simulink model "final_output"  (R2024a)
settings: Solver=VariableStepAuto  StartTime=0.0  StopTime=2  MaxStep=1e-3  RelTol=1e-3  EnableMultiTasking=on
PreLoadFcn:
  | DualActiveBridgeConverterData
values from neighbouring files (symbols this model uses):
  C_HV = 0.0001    [matlab.mat]
  C_LV = 0.002    [matlab.mat]
  Cs_FET = inf    [matlab.mat]
  Fsw = 100000    [matlab.mat]
  Ki_Ireg = 500    [matlab.mat]
  Kp_Ireg = 0.1    [matlab.mat]
  L_Inductor = 1.5e-05    [matlab.mat]
  Lm_Tr = 0.00072    [matlab.mat]
  Lprim_Tr = 1.7e-05    [matlab.mat]
  Lsec_Tr = 0    [matlab.mat]
  N_Tr = 1.6    [matlab.mat]
  Pnom = 10000    [matlab.mat]
  R_DCsrc1 = 0.01    [matlab.mat]
  R_DCsrc2 = 0.05    [matlab.mat]
  R_Inductor = 0.016    [matlab.mat]
  RC_HV = 0.001    [matlab.mat]
  RC_LV = 0.001    [matlab.mat]
  Rm_Tr = 10000    [matlab.mat]
  Ron_Diode = 0.01    [matlab.mat]
  Ron_FET = 0.016    [matlab.mat]
  Rprim_Tr = 0.043    [matlab.mat]
  Rs_FET = 1000000    [matlab.mat]
  Rsec_Tr = 1e-06    [matlab.mat]
  Ts_Control = 1e-06    [matlab.mat]
  Vf_Diode = 4.2    [matlab.mat]
  Vnom_HV = 800    [matlab.mat]
  Vnom_LV = 450    [matlab.mat]
undefined symbols (not defined in the file or in its folder): DiscIntNeverNeededParam, Ion, Lithium
libraries: spsSeriesRLCBranchLib x14, spsDiodeLib x12, spsVoltageMeasurementLib x11, spsMosfetLib x9, spsCurrentMeasurementLib x8, spsIdealSwitchLib x8, powerlib_extras x5, spsMeanLib x5, spsRMSLib x3, simulink x3, spsThreePhaseVIMeasurementLib x2, spsUniversalBridgeLib x2
(part 1 of 2)
settings Model: SimulationMode=accelerator  Creator=The MathWorks, Inc.  LastModifiedBy=suchi
settings SolverCC: ZeroCrossAlgorithm=Adaptive  AlgebraicLoopSolver=TrustRegion
settings DataIOCC: LimitDataPoints=on  SaveFormat=Array  SaveOutput=off  DSMLogging=off  SaveTime=off  ReturnWorkspaceOutputs=off
settings OptimizationCC: LifeSpan=inf
settings DebuggingCC: SaveWithParameterizedLinksMsg=none  UnderspecifiedInitializationDetection=Classic  MergeDetectMultiDrivingBlocksExec=none  IgnoredZcDiagnostic=none  SolverPrmCheckMsg=warning  FcnCallInpInsideContextMsg=warning  UnconnectedInputMsg=warning  UnconnectedOutputMsg=warning  UnconnectedLineMsg=warning  StateNameClashWarn=warning  SubsystemReferenceDiagnosticForUnitTest=warning  SFUnexpectedBacktrackingDiag=warning  SFNoUnconditionalDefaultTransitionDiag=warning  SFExecutionAtInitializationDiag=none  ArithmeticOperatorsInVariantConditions=warning
settings HardwareCC: ProdBitPerPointer=32  ProdBitPerSizeT=32  ProdBitPerPtrDiffT=32  ProdLargestAtomicFloat=None  ProdIntDivRoundTo=Undefined  ProdEndianess=Unspecified  ProdWordSize=32  ProdHWDeviceType=32-bit Generic  TargetHWDeviceType=32-bit Generic
settings ModelReferenceCC: EnableRefExpFcnMdlSchedulingChecks=on  PropagateSignalLabelsOutOfModel=off
settings SFSimCC: SimUseLocalCustomCode=off  CustomCodeUndefinedFunction=UseInterfaceOnly
settings RTWCC: RTWUseLocalCustomCode=off  GPUComputeCapability=3.5  DLArmComputeVersion=19.05
settings CodeAppCC: StateflowObjectComments=on
settings GRTTargetCC: TargetFcnLib=ansi_tfl_tmw.mat  TargetLangStandard=C89/C90 (ANSI)  CombineOutputUpdateFcns=off  GRTInterface=on
settings ConfigComp: CovMetricSettings=dw  CovSaveCumulativeToWorkspaceVar=on  CovSaveSingleToWorkspaceVar=on  CovExternalEMLEnable=off  CovSFcnEnable=off

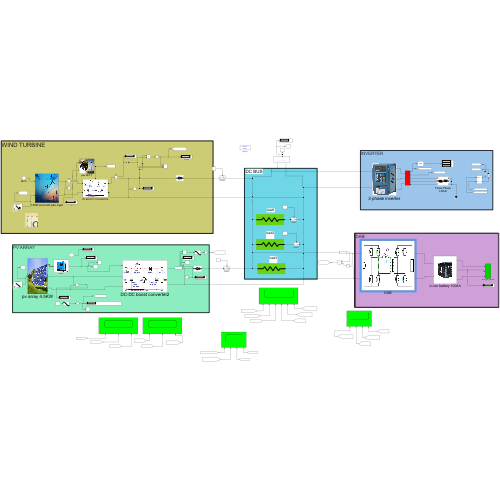
[thumbnail: Simulink's stored preview of the top-level diagram]
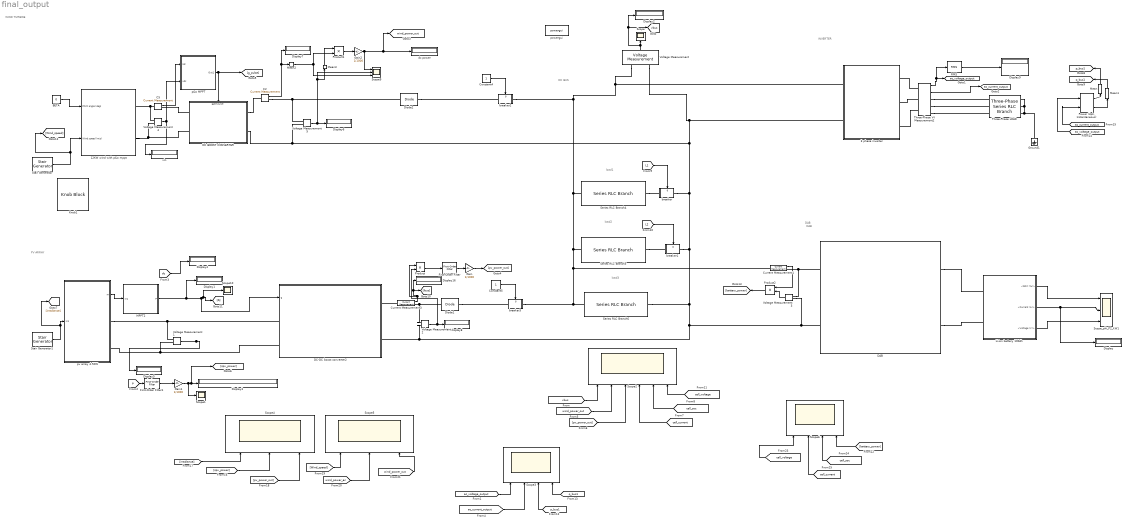
== system final_output ==
  note: DC BUS
  note: load1
  note: INVERTER
  note: DAB
  note: WIND TURBINE
  note: PV ARRAY
  note: load3
  note: load2
  note: DAB
  12KW wind with p&o mppt : Subsystem
      mask Display: image('download (1) - Copy.jpeg');
  3 phase inverter : Subsystem
      mask Display: image('63494ce6710fec25d6700b0f-vfd-inverter-ac-380v-4kw-three-phase.jpg');
  BETA : Constant  Value=0
  C2 : spsCurrentMeasurementLib/Current Measurement  PhasorSimulation=off  OutputType=Complex  PSBequivalent=0
  C5 : spsCurrentMeasurementLib/Current Measurement  PhasorSimulation=off  OutputType=Complex  PSBequivalent=0
  Constant4 : Constant
  Constant5 : Constant
  Current Measurement1 : spsCurrentMeasurementLib/Current Measurement  PhasorSimulation=off  OutputType=Complex  PSBequivalent=0
  Current Measurement3 : spsCurrentMeasurementLib/Current Measurement  PhasorSimulation=off  OutputType=Complex  PSBequivalent=0
  DAB : Subsystem
      mask Display: image('DAB.jpg');
  DC BOOST CONVERTER : Subsystem
      settings: PortSchema="{\"entries\":[{\"content\":{\"sides\":[{\"content\":{\"connectorIds\":[\"LConn1\",\"LConn2\"]},\"type\":\"ConnectorPlacement.EquallySpacedRectSide\",\"uuid\":\"56be2a4d-d0e9-492c-96c1-3864bac83254\"},{\"content\":{\"connectorIds\":[\"RConn1\",\"RConn2\"],\"side\":\"RIGHT\"},\"type\":\"ConnectorPlacement.EquallySpacedRectSide\",\"uuid\":\"94a95191-bdc4-49b6-9a1b-7d416a9cf8d0\"},{\"content\":{\"connectorIds\":[\"In1\"],\"side\":\"TOP\"},\"type\":\"ConnectorPlacement.EquallySpacedRectSide\",\"uuid\":\"679d3c69-2a7c-41fc-a2c8-ece2ac62cc84\"}]},\"type\":\"ConnectorPlacement.EquallySpacedConnector\",\"uuid\":\"33c0da2b-e95a-43d2-a39b-7409ff7da8a9\"}],\"packageUris\":[\"http://schema.mathworks.com/mf0/Connector/R2020b\"],\"version\":\"1.0\"}"
      mask Display: image('boost-converter-working-model.jpg');
  DC-DC boost converter2 : Subsystem
      mask Display: image('boost-converter-working-model.jpg');
  Diode1 : spsDiodeLib/Diode  Ron=0.001  Lon=0  Vf=0.8  IC=0  UseSnubber=0  Rs=inf  Cs=250e-9  Measurements=off
  Diode2 : spsDiodeLib/Diode  Ron=0.001  Lon=0  Vf=0.8  IC=0  UseSnubber=0  Rs=inf  Cs=250e-9  Measurements=off
  Display{,1..9,16} (11 alike) : Display
  First-Order Filter : spsFirstOrderFilterLib/First-Order Filter  FilterType=Lowpass  Tc=10e-3  Ts=0  Initialize=on  Vac_Init=[0, 0, 60]  Vdc_Init=0  PlotResponse=off  FreqRange="[0,  200,  1]"
  First-Order Filter1 : spsFirstOrderFilterLib/First-Order Filter  FilterType=Lowpass  Tc=10e-3  Ts=0  Initialize=on  Vac_Init=[0, 0, 60]  Vdc_Init=0  PlotResponse=off  FreqRange="[0,  200,  1]"
  Gain : Gain  Gain=1/1000
  Gain1 : Gain  Gain=1/1000
  Gain2 : Gain  Gain=1/1000
  Goto11 : Goto
  Ground1 : spsGroundLib/Ground  LConnTagsString=a
  Knob1 : KnobBlock  ScaleMax=20
  Li-ion battery 100Ah : Subsystem
      mask Display: image('Lion-Adventure-side-2000x2000 (1).png');
  MPPT2 : Subsystem
      mask Display: image('48v-50a-mppt-solar-charge-.png');
  Mean : spsMeanLib/Mean  Freq=50  Vinit=0  Ts=0
  Mean1 : spsMeanLib/Mean  Freq=50  Vinit=0  Ts=0
  Mean2 : spsMeanLib/Mean  Freq=50  Vinit=0  Ts=50e-6
  Mean3 : spsMeanLib/Mean  Freq=50  Vinit=0  Ts=50e-6
  "Power (3ph, Instantaneous)" : spsPower3phInstantaneousLib/Power (3ph, Instantaneous)
  Product : Product
  Product1 : Product
  Product2 : Product
  RMS : spsRMSLib/RMS  TrueRMS=on  Freq=50  RMSInit=120  Ts=0
  Scope : Scope
  Scope1 : Scope
  Scope10 : Scope
  Scope2 : Scope  NumInputPorts=6
  Scope3 : Scope  NumInputPorts=4
  Scope4 : Scope  NumInputPorts=3
  Scope5 : Scope  NumInputPorts=3
  Scope6 : Scope  NumInputPorts=4
  Scope9 : Scope  NumInputPorts=3
  Scope_phi_P2_kW1 : Scope  NumInputPorts=3
  Series RLC Branch4 : spsSeriesRLCBranchLib/Series RLC Branch  LConnTagsString=__new0  RConnTagsString=__new0  BranchType=R  Resistance=100  Inductance=1e-9  SetiL0=off  InitialCurrent=0  Capacitance=10  Setx0=off  InitialVoltage=0  Measurements=None
  Series RLC Branch5 : spsSeriesRLCBranchLib/Series RLC Branch  LConnTagsString=__new0  RConnTagsString=__new0  BranchType=R  Resistance=100  Inductance=1e-9  SetiL0=off  InitialCurrent=0  Capacitance=10  Setx0=off  InitialVoltage=0  Measurements=None
  Series RLC Branch6 : spsSeriesRLCBranchLib/Series RLC Branch  LConnTagsString=__new0  RConnTagsString=__new0  BranchType=R  Resistance=120  Inductance=1e-9  SetiL0=off  InitialCurrent=0  Capacitance=10  Setx0=off  InitialVoltage=0  Measurements=None
  Stair Generator : eeStairGenerator/Stair Generator  LabelModeActiveChoice=Discrete  TimeInput=[0 0.4 0.8 1.2 1.4 1.6 1.8 ]  AmplitudeInput=[12 10 8 6 8 10 6 ]  SampleTime=-1  RepeatPattern=off  OutDataTypeStr=double
      settings: LibrarySourceBlock=ee_sl_lib/General Control/Stair Generator
  Stair Generator1 : eeStairGenerator/Stair Generator  LabelModeActiveChoice=Discrete  TimeInput=[0 0.4 0.8 1.2 1.6 1.8 ]  AmplitudeInput=[1000 800 600 400 200 400]  SampleTime=1e-6  RepeatPattern=off  OutDataTypeStr=double
      settings: LibrarySourceBlock=ee_sl_lib/General Control/Stair Generator
  Three-Phase LOAD : spsThreePhaseSeriesRLCBranchLib/Three-Phase Series RLC Branch  LConnTagsString=A|B|C  RConnTagsString=A|B|C  BranchType=RL  Resistance=100  Inductance=100e-3  Capacitance=1e-6  Measurements=None
  Three-Phase V-I Measurement2 : spsThreePhaseVIMeasurementLib/Three-Phase V-I Measurement  VoltageMeasurement=phase-to-phase  SetLabelV=off  LabelV=Vabc  Vpu=off  VpuLL=off  CurrentMeasurement=yes  SetLabelI=off  LabelI=Iabc  Ipu=off  Pbase=100e6  Vbase=500e3  OutputType=Complex  PhasorSimulation=off  PSBequivalent=0
  Voltage Measurement{,1..5} (6 alike) : spsVoltageMeasurementLib/Voltage Measurement  PhasorSimulation=off  OutputType=Complex  PSBequivalent=0
  breaker : Subsystem
      settings: PortSchema="{\"entries\":[{\"content\":{\"sides\":[{\"content\":{\"connectorIds\":[\"LConn1\"]},\"type\":\"ConnectorPlacement.EquallySpacedRectSide\",\"uuid\":\"d9a674fe-e63c-428a-8f68-a3d0edc2d0cb\"},{\"content\":{\"connectorIds\":[\"RConn1\"],\"side\":\"RIGHT\"},\"type\":\"ConnectorPlacement.EquallySpacedRectSide\",\"uuid\":\"8621f35b-529d-46ae-a8cf-f4891c99fec3\"},{\"content\":{\"connectorIds\":[\"In1\"],\"side\":\"TOP\"},\"type\":\"ConnectorPlacement.EquallySpacedRectSide\",\"uuid\":\"fecd911f-8796-40e3-a2af-44f182b78dc1\"}]},\"type\":\"ConnectorPlacement.EquallySpacedConnector\",\"uuid\":\"73397587-ab48-451b-aa61-cf3e3594506e\"}],\"packageUris\":[\"http://schema.mathworks.com/mf0/Connector/R2020b\"],\"version\":\"1.0\"}"
  breaker1 : Subsystem
      settings: PortSchema="{\"entries\":[{\"content\":{\"sides\":[{\"content\":{\"connectorIds\":[\"LConn1\"]},\"type\":\"ConnectorPlacement.EquallySpacedRectSide\",\"uuid\":\"d9a674fe-e63c-428a-8f68-a3d0edc2d0cb\"},{\"content\":{\"connectorIds\":[\"RConn1\"],\"side\":\"RIGHT\"},\"type\":\"ConnectorPlacement.EquallySpacedRectSide\",\"uuid\":\"8621f35b-529d-46ae-a8cf-f4891c99fec3\"},{\"content\":{\"connectorIds\":[\"In1\"],\"side\":\"TOP\"},\"type\":\"ConnectorPlacement.EquallySpacedRectSide\",\"uuid\":\"fecd911f-8796-40e3-a2af-44f182b78dc1\"},{\"content\":{\"side\":\"BOTTOM\"},\"type\":\"ConnectorPlacement.EquallySpacedRectSide\",\"uuid\":\"1105760b-ea89-4923-b494-35b0f35b7535\"}]},\"type\":\"ConnectorPlacement.EquallySpacedConnector\",\"uuid\":\"73397587-ab48-451b-aa61-cf3e3594506e\"}],\"packageUris\":[\"http://schema.mathworks.com/mf0/Connector/R2020b\"],\"version\":\"1.0\"}"
  breaker2 : Subsystem
      settings: PortSchema="{\"entries\":[{\"content\":{\"sides\":[{\"content\":{\"connectorIds\":[\"LConn1\"]},\"type\":\"ConnectorPlacement.EquallySpacedRectSide\",\"uuid\":\"d9a674fe-e63c-428a-8f68-a3d0edc2d0cb\"},{\"content\":{\"connectorIds\":[\"RConn1\"],\"side\":\"RIGHT\"},\"type\":\"ConnectorPlacement.EquallySpacedRectSide\",\"uuid\":\"8621f35b-529d-46ae-a8cf-f4891c99fec3\"},{\"content\":{\"connectorIds\":[\"In1\"],\"side\":\"TOP\"},\"type\":\"ConnectorPlacement.EquallySpacedRectSide\",\"uuid\":\"fecd911f-8796-40e3-a2af-44f182b78dc1\"}]},\"type\":\"ConnectorPlacement.EquallySpacedConnector\",\"uuid\":\"73397587-ab48-451b-aa61-cf3e3594506e\"}],\"packageUris\":[\"http://schema.mathworks.com/mf0/Connector/R2020b\"],\"version\":\"1.0\"}"
  breaker3 : Subsystem
      settings: PortSchema="{\"entries\":[{\"content\":{\"sides\":[{\"content\":{\"connectorIds\":[\"LConn1\"]},\"type\":\"ConnectorPlacement.EquallySpacedRectSide\",\"uuid\":\"d9a674fe-e63c-428a-8f68-a3d0edc2d0cb\"},{\"content\":{\"connectorIds\":[\"RConn1\"],\"side\":\"RIGHT\"},\"type\":\"ConnectorPlacement.EquallySpacedRectSide\",\"uuid\":\"8621f35b-529d-46ae-a8cf-f4891c99fec3\"},{\"content\":{\"connectorIds\":[\"In1\"],\"side\":\"TOP\"},\"type\":\"ConnectorPlacement.EquallySpacedRectSide\",\"uuid\":\"fecd911f-8796-40e3-a2af-44f182b78dc1\"}]},\"type\":\"ConnectorPlacement.EquallySpacedConnector\",\"uuid\":\"73397587-ab48-451b-aa61-cf3e3594506e\"}],\"packageUris\":[\"http://schema.mathworks.com/mf0/Connector/R2020b\"],\"version\":\"1.0\"}"
  dc power : Display
  p&o MPPT : Subsystem
      mask Display: image('Wind-Turbine-MPPT-Charge-Controller (1).png');
  powergui : sps_lib/powergui  Priority=1  SimulationMode=Discrete  SampleTime=1e-6  frequency=60  Iterations=50  frequencyindice=0  Pbase=100e6  ErrMax=1e-4  UnitsV=kV  UnitsW=MW  buscounter=0  FunctionMessages=off  echomessages=off  EnableUseOfTLC=off  CurrentSourceSwitches=off  DisableSnubberDevices=off  DisableRonSwitches=off  DisableVfSwitches=off  DisplayEquations=off  AutomaticDiscreteSolvers=off  SolverType=Tustin/Backward Euler (TBE)  Interpol=off  ExternalGateDelay=off  methode=off  Ts=100  x0status=blocks  SPID=on  SwTol=0  HookPort=off  NonlinearTolerance=1e-4  nMaxIteration=100  ContinueOnMaxIteration=off  RestoreLinks=warning  ResistiveCurrentMeasurement=off  Frange=[0:2:500]  Ylog=off  Xlog=on  ShowGrid=off  save=off  variable=ZData  structure=0  ZoomFFT=off  StartTime=0.0  cycles=1  DisplayStyle=1  fundamental=60  FreqAxis=off  MaxFrequency=1000  frequencyindicesteady=1  RmsSteady=1  display=off
  pv array 4.5KW : Subsystem
      mask Display: image('shutterstock-630302630-solar-panel-dealers-2-i44i3.png');
  vin : Display
  tag scope: ac_current_output=global, ac_voltage_output=global, p_bus1=global, q_bus1=global, vbus=global, wind_power_out=global
  wires:
  Stair Generator1/1 -> [irradiance], pv array 4.5KW/1(In1)
  pv array 4.5KW/1(m) -> MPPT2/1(In1)
  MPPT2/1(P) -> Display1/1, Goto11/1, Scope10/1, DC-DC boost converter2/1(g)
  Current Measurement3/1 -> Product/1, Display16/1, [ibus]
  [dc] -> Display4/1
  Voltage Measurement1/1 -> Display5/1
  RMS/1 -> Display9/1
  Three-Phase V-I Measurement2/1 -> RMS/1, [ac_voltage_output]
  Three-Phase V-I Measurement2/2 -> [ac_current_output]
  [L1] -> breaker/1(g)
  [L2] -> breaker1/1(g)
  Li-ion battery 100Ah/2(<Current (A)>) -> Display/1, Scope_phi_P2_kW1/2
  Li-ion battery 100Ah/1(<SOC (%)>) -> Scope_phi_P2_kW1/1
  Li-ion battery 100Ah/3(<Voltage (V)>) -> Scope_phi_P2_kW1/3
  Voltage Measurement/1 -> [vbus], Display2/1, Scope/1
  BETA/1 -> 12KW wind with p&o mppt/1(Pitch angle (deg))
  Voltage Measurement5/1 -> Display6/1, Mean3/1, Scope9/2
  Mean3/1 -> Product1/1
  Gain2/1 -> Scope9/1, [wind_power_out], dc power/1
  Mean2/1 -> Product1/2, Scope9/3
  C2/1 -> Display7/1, Mean2/1
  Product1/1 -> Gain2/1
  Voltage Measurement2/1 -> Product/2, Display8/1
  [vbus] -> Scope2/1
  [wind_power_out] -> Scope2/2
  Product/1 -> First-Order Filter/1
  [pv_power_out] -> Scope2/3
  Constant4/1 -> breaker2/1(g)
  Constant5/1 -> breaker3/1(g)
  First-Order Filter/1 -> Gain/1
  p&o MPPT/1(Out1) -> [g_pulse], DC BOOST CONVERTER/1(gate pulse)
  Voltage Measurement4/1 -> vin/1, p&o MPPT/2(vdc)
  C5/1 -> p&o MPPT/1(Idc)
  Gain/1 -> [pv_power_out]
  [p] -> First-Order Filter1/1
  First-Order Filter1/1 -> Gain1/1
  Gain1/1 -> Scope1/1, [spv_power], Display3/1
  [cell_current] -> Scope2/4
  [cell_soc] -> Scope2/5
  [cell_voltage] -> Scope2/6
  [ac_voltage_output] -> Scope3/1
  [ac_current_output] -> Scope3/2
  [p_bus1] -> Scope3/3
  [q_bus1] -> Scope3/4
  [ac_voltage_output] -> "Power (3ph, Instantaneous)"/1
  [ac_current_output] -> "Power (3ph, Instantaneous)"/2
  "Power (3ph, Instantaneous)"/1 -> Mean/1
  "Power (3ph, Instantaneous)"/2 -> Mean1/1
  Mean/1 -> [p_bus1]
  Mean1/1 -> [q_bus1]
  [irradiance] -> Scope4/1
  [spv_power] -> Scope4/2
  [pv_power_out] -> Scope4/3
  Stair Generator/1 -> [Wind_speed], 12KW wind with p&o mppt/2(Wind speed (m/s))
  [Wind_speed] -> Scope5/1
  [wind_power_ac] -> Scope5/2
  [wind_power_out] -> Scope5/3
  Voltage Measurement3/1 -> Product2/2
  Current Measurement1/1 -> Product2/1
  Product2/1 -> [battery_power]
  [cell_voltage] -> Scope6/1
  [battery_power] -> Scope6/4
  [cell_soc] -> Scope6/3
  [cell_current] -> Scope6/2
  connections:
  Current Measurement3/RConn1 -- Voltage Measurement2/LConn1 -- Diode1/LConn1
  DC-DC boost converter2/LConn2 -- Voltage Measurement1/LConn2 -- pv array 4.5KW/RConn2
  pv array 4.5KW/RConn1 -- Voltage Measurement1/LConn1 -- DC-DC boost converter2/LConn1
  Current Measurement3/LConn1 -- DC-DC boost converter2/RConn1
  Three-Phase LOAD/RConn1 -- Ground1/LConn1 -- Three-Phase LOAD/RConn3 -- Three-Phase LOAD/RConn2
  Three-Phase V-I Measurement2/LConn3 -- 3 phase inverter/LConn3
  Three-Phase V-I Measurement2/LConn1 -- 3 phase inverter/LConn1
  Three-Phase V-I Measurement2/RConn1 -- Three-Phase LOAD/LConn1
  Three-Phase V-I Measurement2/LConn2 -- 3 phase inverter/LConn2
  DAB/LConn1 -- Voltage Measurement3/LConn1 -- Current Measurement1/RConn1
  Series RLC Branch4/RConn1 -- breaker/LConn1
  Series RLC Branch5/RConn1 -- breaker1/LConn1
  DAB/RConn1 -- Li-ion battery 100Ah/LConn1
  DAB/RConn2 -- Li-ion battery 100Ah/LConn2
  Voltage Measurement5/LConn2 -- DC BOOST CONVERTER/RConn2 -- Voltage Measurement/LConn2 -- 3 phase inverter/RConn2 -- Voltage Measurement3/LConn2 -- DAB/LConn2 -- DC-DC boost converter2/RConn2 -- Voltage Measurement2/LConn2 -- Series RLC Branch6/RConn1 -- breaker1/RConn1 -- breaker/RConn1
  C2/RConn1 -- Voltage Measurement5/LConn1 -- Diode2/LConn1
  Diode2/RConn1 -- breaker2/LConn1
  Diode1/RConn1 -- breaker3/LConn1
  DC BOOST CONVERTER/RConn1 -- C2/LConn1
  12KW wind with p&o mppt/RConn2 -- Voltage Measurement4/LConn2 -- DC BOOST CONVERTER/LConn2
  C5/LConn1 -- Voltage Measurement4/LConn1 -- 12KW wind with p&o mppt/RConn1
  C5/RConn1 -- DC BOOST CONVERTER/LConn1
  Three-Phase V-I Measurement2/RConn2 -- Three-Phase LOAD/LConn2
  Three-Phase V-I Measurement2/RConn3 -- Three-Phase LOAD/LConn3
  Current Measurement1/LConn1 -- breaker3/RConn1 -- Series RLC Branch6/LConn1 -- Voltage Measurement/LConn1 -- 3 phase inverter/RConn1 -- breaker2/RConn1 -- Series RLC Branch4/LConn1 -- Series RLC Branch5/LConn1

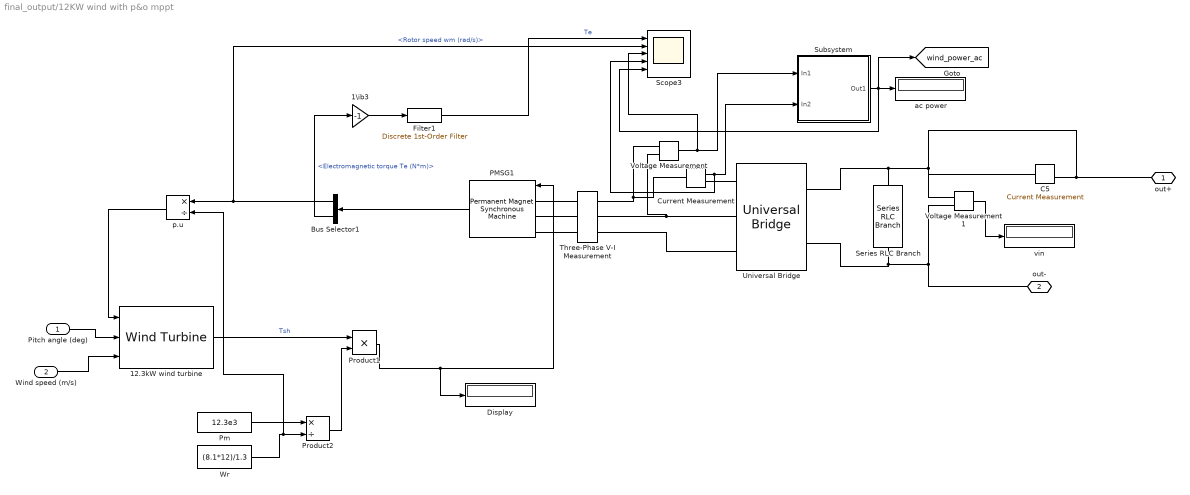
== system final_output/12KW wind with p&o mppt ==
  Pitch angle (deg) : Inport
  Wind speed (m/s) : Inport  Port=2
  "12.3kW wind turbine " : spsWindTurbineLib/Wind Turbine  Pnom=12.3e3  Pelec_base=12.3e3/0.9  wind_base=12  P_wind_base=0.85  speed_nom=1.2  pitch_angle=0  c1_c6="[0.51763          116          0.4            5           21     0.006795]"  cp_nom=0.48  lambda_nom=8.1
  1\ib3 : Gain  Gain=-1  SaturateOnIntegerOverflow=on  OutDataTypeStr=Inherit: Same as input  ParamDataTypeStr=Inherit: Same as input
  Bus Selector1 : BusSelector  OutputSignals=Rotor speed wm (rad/s),Electromagnetic torque Te (N*m)
  C5 : spsCurrentMeasurementLib/Current Measurement  PhasorSimulation=off  OutputType=Complex  PSBequivalent=0
  Current Measurement : spsCurrentMeasurementLib/Current Measurement  PhasorSimulation=off  OutputType=Complex  PSBequivalent=0
  Display : Display
  Filter1 : powerlib_extras/Discrete  Control Blocks/Discrete 1st-Order Filter  FilterType=Lowpass  Tc=1e-3  Ts=50e-6  Initialize=off  Vac_Init=[0.8 -25 50]  Vdc_Init=-0.4  PlotResponse=off  param1=[1 500 0.1]
  PMSG1 : spsPermanentMagnetSynchronousMachineLib/Permanent Magnet Synchronous Machine  NbPhases=3  FluxDistribution=Sinusoidal  RotorType=Salient-pole  MechanicalLoad=Torque Tm  PresetModel=No  ShowDetailedParameters=on  MeasurementBus=off  Resistance=0.0485  Inductance=8.5e-3  dqInductances=[0.395e-3 0.395e-3]  La=0.000835  MachineConstant=Flux linkage established by magnets (V.s)  Flux=0.1194  VoltageCst=108.2838  TorqueCst=0.8955  Flat=120  Mechanical=[0.01197 0.001189 5]  PolePairs=5  InitialConditions=[0,0, 0,0]  InitialConditions5ph=[0 0 0 0 0 0]  RefAngle=90 degrees behind phase A axis (modified Park)  IterativeDiscreteModel=Trapezoidal non iterative  TsBlock=-1  TsPowergui=0
  Pm : Constant  Value=12.3e3
  Product1 : Product
  Product2 : Product  Inputs=*/
  Scope3 : Scope  NumInputPorts=5
  Series RLC Branch : spsSeriesRLCBranchLib/Series RLC Branch  LConnTagsString=__new0  RConnTagsString=__new0  BranchType=RC  Resistance=0.005  Inductance=1e-3  SetiL0=off  InitialCurrent=0  Capacitance=6.60937e-03  Setx0=off  InitialVoltage=0  Measurements=None
  Subsystem : Subsystem
  Three-Phase V-I Measurement : spsThreePhaseVIMeasurementLib/Three-Phase V-I Measurement  VoltageMeasurement=no  SetLabelV=off  LabelV=Vabc  Vpu=off  VpuLL=off  CurrentMeasurement=no  SetLabelI=off  LabelI=Iabc  Ipu=off  Pbase=100e6  Vbase=500e3  OutputType=Complex  PhasorSimulation=off  PSBequivalent=0
  Universal Bridge : spsUniversalBridgeLib/Universal Bridge  Arms=3  SnubberResistance=1e5  SnubberCapacitance=inf  Device=Diodes  Ron=1e-3  Lon=0  ForwardVoltages="[  0  0  ]"  ForwardVoltage=0  GTOparameters=[ 10e-6 , 20e-6 ]  IGBTparameters=[ 1e-6 , 2e-6 ]  Measurements=None  Measurements_2=None  converterType=Rectifier
  Voltage Measurement : spsVoltageMeasurementLib/Voltage Measurement  PhasorSimulation=off  OutputType=Complex  PSBequivalent=0
  Voltage Measurement1 : spsVoltageMeasurementLib/Voltage Measurement  PhasorSimulation=off  OutputType=Complex  PSBequivalent=0
  Wr : Constant  Value=(8.1*12)/1.3
  ac power : Display
  p.u : Product  Inputs=*/
  vin : Display
  out+ : PMIOPort  Side=Right
  out- : PMIOPort  Port=2  Side=Right
  tag scope: wind_power_ac=global
  wires:
  Voltage Measurement/1 -> Scope3/3, Subsystem/1(In1)
  PMSG1/1 -> Bus Selector1/1
  Wr/1 -> p.u/2, Product2/2
  Bus Selector1/1 -> Scope3/2, p.u/1  "<Rotor speed wm (rad/s)>"
  Pm/1 -> Product2/1
  p.u/1 -> "12.3kW wind turbine "/1
  Filter1/1 -> Scope3/1  "Te"
  1\ib3/1 -> Filter1/1
  Subsystem/1(Out1) -> [wind_power_ac], Scope3/5, ac power/1
  Voltage Measurement1/1 -> vin/1
  Product1/1 -> PMSG1/1, Display/1
  Product2/1 -> Product1/2
  Bus Selector1/2 -> 1\ib3/1  "<Electromagnetic torque Te (N*m)>"
  Current Measurement/1 -> Scope3/4, Subsystem/2(In2)
  "12.3kW wind turbine "/1 -> Product1/1  "Tsh"
  Pitch angle (deg)/1 -> "12.3kW wind turbine "/2
  Wind speed (m/s)/1 -> "12.3kW wind turbine "/3
  connections:
  PMSG1/LConn2 -- Three-Phase V-I Measurement/LConn2
  C5/RConn1 -- out+/RConn1 -- Universal Bridge/RConn1 -- Series RLC Branch/LConn1 -- Voltage Measurement1/LConn1 -- C5/LConn1
  Voltage Measurement/LConn1 -- Three-Phase V-I Measurement/RConn1 -- Current Measurement/LConn1
  Three-Phase V-I Measurement/RConn3 -- Universal Bridge/LConn3
  PMSG1/LConn3 -- Three-Phase V-I Measurement/LConn3
  Current Measurement/RConn1 -- Universal Bridge/LConn1
  PMSG1/LConn1 -- Three-Phase V-I Measurement/LConn1
  Voltage Measurement/LConn2 -- Universal Bridge/LConn2 -- Three-Phase V-I Measurement/RConn2
  Voltage Measurement1/LConn2 -- out-/RConn1 -- Universal Bridge/RConn2 -- Series RLC Branch/RConn1

== system final_output/3 phase inverter ==
  Demux : Demux  Outputs=6
  PWM Generator (2-Level) : spsPWMGenerator2LevelLib/PWM Generator (2-Level)  ModulatorType=Three-phase bridge (6 pulses)  ModulatorMode=Unsynchronized  Fc=1000  Pc=90  nF=27  MinMax="[ -1  1 ]"  SamplingTechnique=Natural  ModulatingSignals=on  m=0.5  Freq=50  Phase=0  Ts=0  ShowCarrierOutport=off
  Scope : Scope  NumInputPorts=6
  Universal Bridge : spsUniversalBridgeLib/Universal Bridge  Arms=3  SnubberResistance=1e5  SnubberCapacitance=inf  Device=MOSFET / Diodes  Ron=1e-3  Lon=0  ForwardVoltages="[  0  0  ]"  ForwardVoltage=0  GTOparameters=[ 10e-6 , 20e-6 ]  IGBTparameters=[ 1e-6 , 2e-6 ]  Measurements=None  Measurements_2=None  converterType=Rectifier
  A : PMIOPort  Side=Left
  + : PMIOPort  Port=2  Side=Right
  B : PMIOPort  Port=3  Side=Left
  - : PMIOPort  Port=4  Side=Right
  C : PMIOPort  Port=5  Side=Left
  wires:
  PWM Generator (2-Level)/1 -> Universal Bridge/1, Demux/1
  Demux/1 -> Scope/1
  Demux/2 -> Scope/2
  Demux/3 -> Scope/3
  Demux/4 -> Scope/4
  Demux/5 -> Scope/5
  Demux/6 -> Scope/6
  connections:
  A/RConn1 -- Universal Bridge/LConn1
  -/RConn1 -- Universal Bridge/RConn2
  B/RConn1 -- Universal Bridge/LConn2
  C/RConn1 -- Universal Bridge/LConn3
  +/RConn1 -- Universal Bridge/RConn1

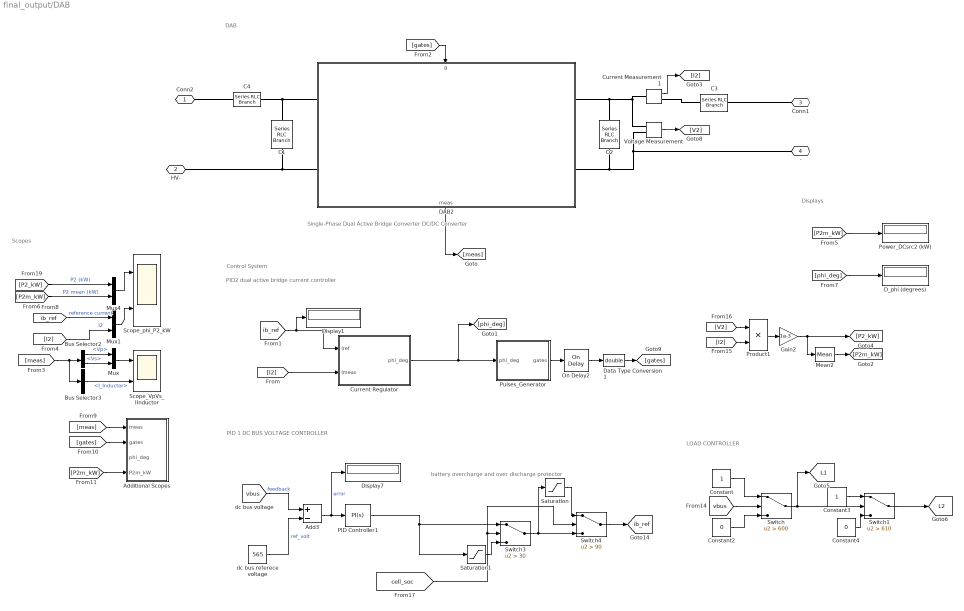
== system final_output/DAB ==
  note: DAB
  note: LOAD CONTROLLER
  note: battery overcharge and over discharge protector
  note: PID 1 DC BUS VOLTAGE CONTROLLER
  note: PID2 dual active bridge current controller
  note: Single-Phase Dual Active Bridge Converter DC/DC Converter
  note: Control System
  note: Scopes
  note: Displays
  Add3 : Sum  Inputs=+-
  Additional Scopes : Subsystem
  Bus Selector2 : BusSelector  OutputSignals=Vp,Vs
  Bus Selector3 : BusSelector  OutputSignals=I_Inductor
  C1 : spsSeriesRLCBranchLib/Series RLC Branch  LConnTagsString=__new0  RConnTagsString=__new0  BranchType=RC  Resistance=RC_HV  Inductance=1  SetiL0=off  InitialCurrent=0  Capacitance=C_HV  Setx0=off  InitialVoltage=0  Measurements=None
  C2 : spsSeriesRLCBranchLib/Series RLC Branch  LConnTagsString=__new0  RConnTagsString=__new0  BranchType=RC  Resistance=RC_LV  Inductance=1  SetiL0=off  InitialCurrent=0  Capacitance=C_LV  Setx0=off  InitialVoltage=0  Measurements=None
  C3 : spsSeriesRLCBranchLib/Series RLC Branch  LConnTagsString=__new0  RConnTagsString=__new0  BranchType=R  Resistance=R_DCsrc2  Inductance=100e-6  SetiL0=off  InitialCurrent=0  Capacitance=1  Setx0=off  InitialVoltage=0  Measurements=None
  C4 : spsSeriesRLCBranchLib/Series RLC Branch  LConnTagsString=__new0  RConnTagsString=__new0  BranchType=R  Resistance=R_DCsrc1  Inductance=1  SetiL0=off  InitialCurrent=0  Capacitance=1  Setx0=off  InitialVoltage=0  Measurements=None
  Constant : Constant
  Constant2 : Constant  Value=0
  Constant3 : Constant
  Constant4 : Constant  Value=0
  Current Measurement1 : spsCurrentMeasurementLib/Current Measurement  PhasorSimulation=off  OutputType=Complex  PSBequivalent=0
  Current Regulator : Subsystem
  DAB2 : Subsystem  mask(Single-phase, Dual-Active Bridge DC/DC Converter){Ron_FET=Ron_FET, RsCs_FET=[Rs_FET, Cs_FET], Ron_Diode=Ron_Diode, Vf_Diode=Vf_Diode, RL_Inductor=[R_Inductor, L_Inductor], Param1_Tr=[Pnom, Fsw], Param2_Tr=[Vnom_HV, Rprim_Tr, Lprim_Tr], Param3_Tr=[Vnom_HV/N_Tr, Rsec_Tr, Lsec_Tr], Param4_Tr=[Rm_Tr, Lm_Tr]}
      mask prompts: Ron_FET "Ron FET"; RsCs_FET "FET snubber: [Rs (ohm)  Cs (F)]"; RL_Inductor "Coupling inductor [ R (ohms)   L (H)]"; Param1_Tr "Nominal power and frequency [Pn(VA) fn(Hz)]:"; Param2_Tr "Winding 1 parameters [V1(Vrms) R1(ohm) L1(H)]:"; Param3_Tr "Winding 2 parameters [V2(Vrms) R2(ohm) L2(H)]:"; Param4_Tr "Magnetization resistance and inductance [Rm(ohm) Lm(H)]:"
      mask init:
      | Rs_FET=RsCs_FET(1);
      | Cs_FET=RsCs_FET(2);
      | R_Inductor=RL_Inductor(1);
      | L_Inductor=RL_Inductor(2);
      settings: PortSchema="{\"entries\":[{\"content\":{\"sides\":[{\"content\":{\"connectorIds\":[\"LConn1\",\"LConn2\"]},\"type\":\"ConnectorPlacement.EquallySpacedRectSide\",\"uuid\":\"9324ea44-499c-4ecb-9e49-362befe9c555\"},{\"content\":{\"connectorIds\":[\"RConn1\",\"RConn2\"],\"side\":\"RIGHT\"},\"type\":\"ConnectorPlacement.EquallySpacedRectSide\",\"uuid\":\"1d2d188e-4a2f-457a-9d2e-cac68811a3aa\"},{\"content\":{\"connectorIds\":[\"In1\"],\"side\":\"TOP\"},\"type\":\"ConnectorPlacement.EquallySpacedRectSide\",\"uuid\":\"7f41b21e-a624-46b0-bf38-abdafc8e74d0\"},{\"content\":{\"connectorIds\":[\"Out1\"],\"side\":\"BOTTOM\"},\"type\":\"ConnectorPlacement.EquallySpacedRectSide\",\"uuid\":\"ef27d855-3875-49de-80dc-d9576eabadca\"}]},\"type\":\"ConnectorPlacement.EquallySpacedConnector\",\"uuid\":\"30393c4b-568d-4140-9cdd-d3267fa7bc9d\"}],\"packageUris\":[\"http://schema.mathworks.com/mf0/Connector/R2020b\"],\"version\":\"1.0\"}"
      mask Display: image('$imagefile')
  D_phi (degrees) : Display
      settings: Format=bank  Decimation=100
  Data Type Conversion1 : DataTypeConversion  OutDataTypeStr=double  SaturateOnIntegerOverflow=off  RndMeth=Floor
  Display1 : Display
  Display7 : Display
  Gain2 : Gain  Gain=1e-3
  Mean2 : spsMeanLib/Mean  Freq=Fsw  Vinit=0  Ts=0
  Mux : Mux  Inputs=2
  Mux1 : Mux  Inputs=2
  Mux4 : Mux  Inputs=2
  On Delay2 : spsOnDelayLib/On Delay  DelayType=On delay  delay=DT  ic=0  Ts=0
  PID Controller1 : slpidlib/PID Controller  Controller=PI  Form=Parallel  TimeDomain=Continuous-time  UseExternalTs=off  SampleTime=1e-6  IntegratorMethod=Forward Euler  FilterMethod=Forward Euler  ControllerParametersSource=internal  P=0.1  I=60  UseKiTs=off  D=0  UseExternalDerivativeSource=off  N=100  UseFilter=on  TunerSelectOption=Transfer Function Based (PID Tuner App)  InitialConditionSource=internal  InitialConditionForIntegrator=0  InitialConditionForFilter=0  DifferentiatorICPrevScaledInput=0  ExternalReset=none  TrackingMode=off  Kt=1  LimitOutput=on  SatLimitsSource=internal  UpperSaturationLimit=25  LowerSaturationLimit=-25  LinearizeAsGain=on  AntiWindupMode=none  Kb=1  LimitIntegrator=off  UpperIntegratorSaturationLimit=inf  LowerIntegratorSaturationLimit=-inf  POutMin=[]  POutMax=[]  IOutMin=[]  IOutMax=[]  DOutMin=[]  DOutMax=[]  NOutMin=[]  NOutMax=[]  SumOutMin=[]  SumOutMax=[]  SaturationOutMin=[]  SaturationOutMax=[]  PParamMin=[]  PParamMax=[]  IParamMin=[]  IParamMax=[]  DParamMin=[]  DParamMax=[]  NParamMin=[]  NParamMax=[]  KbParamMin=[]  KbParamMax=[]  KtParamMin=[]  KtParamMax=[]  KbOutMin=[]  KbOutMax=[]  KtOutMin=[]  KtOutMax=[]  IntegratorOutMin=[]  IntegratorOutMax=[]  FilterOutMin=[]  FilterOutMax=[]  SumI1OutMin=[]  SumI1OutMax=[]  SumI2OutMin=[]  SumI2OutMax=[]  SumI3OutMin=[]  SumI3OutMax=[]  SumI4OutMin=[]  SumI4OutMax=[]  SumDOutMin=[]  SumDOutMax=[]  DifferentiatorOutMin=[]  DifferentiatorOutMax=[]  FilterDiffOutCoefMin=[]  FilterDiffOutCoefMax=[]  ReciprocalOutMin=[]  ReciprocalOutMax=[]  SumDenOutMin=[]  SumDenOutMax=[]  SumNumOutMin=[]  SumNumOutMax=[]  DivideOutMin=[]  DivideOutMax=[]  UdiffTsProdOutMin=[]  UdiffTsProdOutMax=[]  NTsProdOutMin=[]  NTsProdOutMax=[]  UintegralTsProdOutMin=[]  UintegralTsProdOutMax=[]  UngainTsProdOutMin=[]  UngainTsProdOutMax=[]  ClampingZeroOutDataTypeStr=Inherit: Inherit via back propagation  ClampingZeroOutMin=[]  ClampingZeroOutMax=[]  FilterDenConstantOutDataTypeStr=Inherit: Inherit via back propagation  FilterDenConstantOutMin=[]  FilterDenConstantOutMax=[]  PCopyOutDataTypeStr=Inherit: Inherit via back propagation  PCopyOutMin=[]  PCopyOutMax=[]  NCopyOutDataTypeStr=Inherit: Inherit via back propagation  NCopyOutMin=[]  NCopyOutMax=[]  IntegratorContinuousStateAttributes=''  IntegratorStateMustResolveToSignalObject=off  IntegratorRTWStateStorageClass=Auto  FilterContinuousStateAttributes=''  FilterStateMustResolveToSignalObject=off  FilterRTWStateStorageClass=Auto  ParallelPVariant=InternalParameters  IdealPVariant=Disabled  IVariant=InternalParameters  DVariant=Disabled  IntegratorVariant=Continuous  SatVariant=Enabled  AWVariant=Passthrough  PCopyVariant=Disabled  TRVariant=Disabled  FdbkBlocksVariant=Forward  IdealPFdbkVariant=Disabled  SatFdbkVariant=Disabled  DerivativeFilterVariant=Disabled  NVariant=Disabled  NCopyVariant=Disabled_SignalSpec  FilterICVariant=Disabled  IntegratorICVariant=InternalICs  ExternalResetVariant=Disabled  TRSumVariant=Passthrough  SumFdbkVariant=Disabled  SumVariant=Sum_PI  TsampFilterVariant=InternalTs  TsampNgainVariant=Passthrough  TsampIntegralVariant=Disabled_SignalSpec  ExternalSaturationOutDataTypeStr=Inherit: Same as second input  DerivativeSourceVariant=Disabled
  Power_DCsrc2 (kW) : Display
      settings: Format=bank  Decimation=100
  Product1 : Product
  Pulses_Generator : Subsystem
  Saturation : Saturate  UpperLimit=0  LowerLimit=-30
  Saturation1 : Saturate  UpperLimit=25  LowerLimit=0
  Scope_VpVs_IInductor : Scope  NumInputPorts=2
  Scope_phi_P2_kW : Scope  NumInputPorts=2
  Switch : Switch  Criteria=u2 > Threshold  Threshold=600  SaturateOnIntegerOverflow=off  InputSameDT=off
  Switch1 : Switch  Criteria=u2 > Threshold  Threshold=610  SaturateOnIntegerOverflow=off  InputSameDT=off
  Switch3 : Switch  Criteria=u2 > Threshold  Threshold=30  SaturateOnIntegerOverflow=off  InputSameDT=off
  Switch4 : Switch  Criteria=u2 > Threshold  Threshold=90  SaturateOnIntegerOverflow=off  InputSameDT=off
  Voltage Measurement : spsVoltageMeasurementLib/Voltage Measurement  PhasorSimulation=off  OutputType=Complex  PSBequivalent=0
  dc bus referece voltage : Constant  Value=565
  Conn2 : PMIOPort  Side=Left
  HV- : PMIOPort  Port=2  Side=Left
  Conn1 : PMIOPort  Port=3  Side=Right
  - : PMIOPort  Port=4  Side=Right
  tag scope: L1=global, L2=global, ib_ref=global
  wires:
  Pulses_Generator/1(gates) -> On Delay2/1
  Bus Selector2/2 -> Mux/2  "<Vs>"
  [P2m_kW] -> Additional Scopes/4(P2m_kW)
  [P2_kW] -> Mux4/1  "P2 (kW)"
  Voltage Measurement/1 -> [V2]
  [I2] -> Mux1/2  "I2"
  Gain2/1 -> Mean2/1, [P2_kW]
  Bus Selector2/1 -> Mux/1  "<Vp>"
  [gates] -> DAB2/1(g)
  [P2m_kW] -> Mux4/2  "P2 mean (kW)"
  [phi_deg] -> D_phi (degrees)/1
  DAB2/1(meas) -> [meas]
  Data Type Conversion1/1 -> [gates]
  [gates] -> Additional Scopes/2(gates)
  Current Measurement1/1 -> [I2]
  Mean2/1 -> [P2m_kW]
  Bus Selector3/1 -> Scope_VpVs_IInductor/2  "<I_Inductor>"
  On Delay2/1 -> Data Type Conversion1/1
  [I2] -> Product1/2
  Mux1/1 -> Scope_phi_P2_kW/2
  [P2m_kW] -> Power_DCsrc2 (kW)/1
  [meas] -> Additional Scopes/1(meas)
  [V2] -> Product1/1
  Product1/1 -> Gain2/1
  [I2] -> Current Regulator/2(Imeas)
  [meas] -> Bus Selector3/1, Bus Selector2/1
  Mux/1 -> Scope_VpVs_IInductor/1
  Current Regulator/1(phi_deg) -> [phi_deg], Pulses_Generator/1(phi_deg)
  Add3/1 -> Display7/1, PID Controller1/1  "error"
  [vbus] -> Add3/1  "feedback"
  dc bus referece voltage/1 -> Add3/2  "ref_volt"
  [ib_ref] -> Current Regulator/1(Iref), Display1/1
  [vbus] -> Switch/2
  Constant/1 -> Switch/1
  Constant2/1 -> Switch/3
  Constant4/1 -> Switch1/3
  Constant3/1 -> Switch1/1
  Switch/1 -> [L1], Switch1/2
  Switch1/1 -> [L2]
  PID Controller1/1 -> Saturation1/1, Switch3/1
  Switch3/1 -> Switch4/3, Saturation/1
  Switch4/1 -> [ib_ref]
  [cell_soc] -> Switch4/2, Switch3/2
  Saturation/1 -> Switch4/1
  Saturation1/1 -> Switch3/3
  [ib_ref] -> Mux1/1  "reference current"
  Mux4/1 -> Scope_phi_P2_kW/1
  connections:
  C2/RConn1 -- Voltage Measurement/LConn1 -- Current Measurement1/LConn1 -- DAB2/RConn1
  C1/LConn1 -- HV-/RConn1 -- DAB2/LConn2
  Current Measurement1/RConn1 -- C3/RConn1
  C4/RConn1 -- Conn2/RConn1
  DAB2/RConn2 -- C2/LConn1 -- Voltage Measurement/LConn2 -- -/RConn1
  DAB2/LConn1 -- C4/LConn1 -- C1/RConn1
  C3/LConn1 -- Conn1/RConn1

== system final_output/DC BOOST CONVERTER ==
  note: dc-dc boost converter
  gate pulse : Inport
  Diode3 : spsDiodeLib/Diode  Ron=0.001  Lon=0  Vf=0.8  IC=0  UseSnubber=0  Rs=500  Cs=250e-9  Measurements=off
  Mosfet1 : spsMosfetLib/Mosfet  Ron=0.1  Lon=0  Rd=0.01  Vfd=0  IC=0  Rs=1e5  Cs=inf  Measurements=off
  Series RLC Branch2 : spsSeriesRLCBranchLib/Series RLC Branch  LConnTagsString=__new0  RConnTagsString=__new0  BranchType=L  Resistance=0.005  Inductance=4.55e-05  SetiL0=off  InitialCurrent=0  Capacitance=6.60937e-04  Setx0=off  InitialVoltage=0  Measurements=None
  Series RLC Branch3 : spsSeriesRLCBranchLib/Series RLC Branch  LConnTagsString=__new0  RConnTagsString=__new0  BranchType=RC  Resistance=0.005  Inductance=1e-3  SetiL0=off  InitialCurrent=0  Capacitance=6.60937e-04  Setx0=off  InitialVoltage=0  Measurements=None
  in+ : PMIOPort  Side=Left
  in- : PMIOPort  Port=2  Side=Left
  out+ : PMIOPort  Port=3  Side=Right
  out- : PMIOPort  Port=4  Side=Right
  wires:
  gate pulse/1 -> Mosfet1/1
  connections:
  in+/RConn1 -- Series RLC Branch2/RConn1
  Series RLC Branch3/LConn1 -- out+/RConn1 -- Diode3/RConn1
  Mosfet1/LConn1 -- Series RLC Branch2/LConn1 -- Diode3/LConn1
  Series RLC Branch3/RConn1 -- Mosfet1/RConn1 -- in-/RConn1 -- out-/RConn1

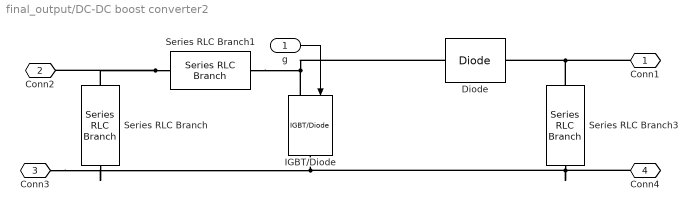
== system final_output/DC-DC boost converter2 ==
  g : Inport
  Diode : spsDiodeLib/Diode  Ron=0.001  Lon=0  Vf=0.8  IC=0  UseSnubber=0  Rs=500  Cs=250e-9  Measurements=off
  IGBT/Diode : spsIGBTDiodeLib/IGBT//Diode  Ron=1e-3  Rs=1e5  Cs=inf  Measurements=off
  Series RLC Branch : spsSeriesRLCBranchLib/Series RLC Branch  LConnTagsString=__new0  RConnTagsString=__new0  BranchType=RC  Resistance=1e-4  Inductance=1e-3  SetiL0=off  InitialCurrent=0  Capacitance=1e-6  Setx0=on  InitialVoltage=0  Measurements=None
  Series RLC Branch1 : spsSeriesRLCBranchLib/Series RLC Branch  LConnTagsString=__new0  RConnTagsString=__new0  BranchType=L  Resistance=0.001  Inductance=0.003  SetiL0=on  InitialCurrent=0  Capacitance=100e-6  Setx0=off  InitialVoltage=0  Measurements=None
  Series RLC Branch3 : spsSeriesRLCBranchLib/Series RLC Branch  LConnTagsString=__new0  RConnTagsString=__new0  BranchType=RC  Resistance=1e-4  Inductance=5e-3  SetiL0=off  InitialCurrent=0  Capacitance=10e-06  Setx0=off  InitialVoltage=0  Measurements=None
  Conn1 : PMIOPort  Side=Right
  Conn2 : PMIOPort  Port=2  Side=Left
  Conn3 : PMIOPort  Port=3  Side=Left
  Conn4 : PMIOPort  Port=4  Side=Right
  wires:
  g/1 -> IGBT/Diode/1
  connections:
  Conn1/RConn1 -- Series RLC Branch3/RConn1 -- Diode/RConn1
  Series RLC Branch1/RConn1 -- Conn2/RConn1 -- Series RLC Branch/LConn1
  Series RLC Branch1/LConn1 -- Diode/LConn1 -- IGBT/Diode/LConn1
  Series RLC Branch3/LConn1 -- Conn4/RConn1 -- Conn3/RConn1 -- Series RLC Branch/RConn1 -- IGBT/Diode/RConn1

== system final_output/Li-ion battery 100Ah ==
  Battery1 : spsBatteryLib/Battery  BatType=Lithium-Ion  ShowTempParam=off  ThermalPreset=no  ShowAgeParam=off  NomV=100  NomQ=100  SOC=50  Batt_Tr=30  PresetModel=on  MaxQ=100  MinV=75  FullV=116.3987  Dis_rate=43.4783  R=0.01  Normal_OP=90.4348  expZone="[108.0386      4.913043]"  current=[6.5 13 32.5]  Units=Time  Tci=20  NomT=20  T2=-30  MaxQ2=4.8  FullV2=7.1  Normal_OP2=5.655  expZone2="[6.58           1]"  Rca=0.6  ti=2000  Dp=0  Neq0=0  Tsim=1e6  Ta1=25  Qeol=5.4*0.9  Reol=0.013333*1.2  Char_age=[2.3478, 3]  Dis_age=[2.3478, 10]  N1=1500  N2=10500  N3=1000  N4=1400  Ta2=45  N5=950
  Bus Selector : BusSelector  OutputSignals=SOC (%),Current (A),Voltage (V)
  + : PMIOPort  Side=Left
  - : PMIOPort  Port=2  Side=Left
  <SOC (%)> : Outport
  <Current (A)> : Outport  Port=2
  <Voltage (V)> : Outport  Port=3
  tag scope: cell_current=global, cell_soc=global, cell_voltage=global
  wires:
  Battery1/1 -> Bus Selector/1
  Bus Selector/3 -> [cell_voltage], <Voltage (V)>/1  "<Voltage (V)>"
  Bus Selector/1 -> [cell_soc], <SOC (%)>/1  "<SOC (%)>"
  Bus Selector/2 -> [cell_current], <Current (A)>/1  "<Current (A)>"
  connections:
  -/RConn1 -- Battery1/LConn2
  +/RConn1 -- Battery1/LConn1

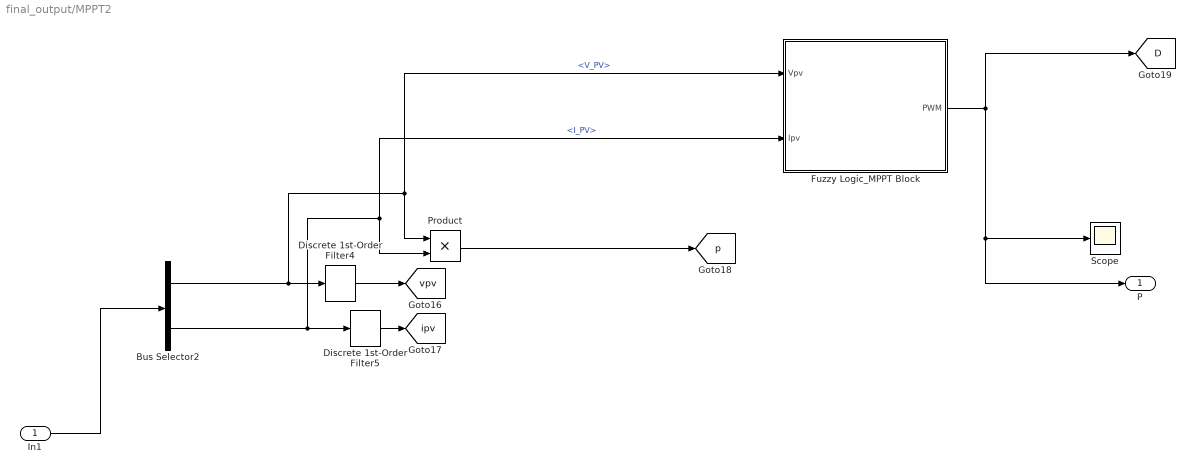
== system final_output/MPPT2 ==
  In1 : Inport
  Bus Selector2 : BusSelector  OutputSignals=V_PV,I_PV
  Discrete 1st-Order Filter4 : powerlib_extras/Discrete  Control Blocks/Discrete 1st-Order Filter  FilterType=Lowpass  Tc=100e-3  Ts=20e-6  Initialize=off  Vac_Init=[0.8 -25 60]  Vdc_Init=-0.4  PlotResponse=off  param1=[1 500 0.1]
  Discrete 1st-Order Filter5 : powerlib_extras/Discrete  Control Blocks/Discrete 1st-Order Filter  FilterType=Lowpass  Tc=100e-3  Ts=20e-6  Initialize=off  Vac_Init=[0.8 -25 60]  Vdc_Init=-0.4  PlotResponse=off  param1=[1 500 0.1]
  Fuzzy Logic_MPPT Block : Subsystem
  Product : Product
  Scope : Scope
  P : Outport
  tag scope: D=global, ipv=global, p=global, vpv=global
  wires:
  Fuzzy Logic_MPPT Block/1(PWM) -> [D], P/1, Scope/1
  In1/1 -> Bus Selector2/1
  Bus Selector2/1 -> Discrete 1st-Order Filter4/1, Product/1, Fuzzy Logic_MPPT Block/1(Vpv)  "<V_PV>"
  Bus Selector2/2 -> Discrete 1st-Order Filter5/1, Product/2, Fuzzy Logic_MPPT Block/2(Ipv)  "<I_PV>"
  Product/1 -> [p]
  Discrete 1st-Order Filter4/1 -> [vpv]
  Discrete 1st-Order Filter5/1 -> [ipv]

== system final_output/breaker ==
  g : Inport
  Mosfet : spsMosfetLib/Mosfet  Ron=0.1  Lon=0  Rd=0.01  Vfd=0  IC=0  Rs=1e5  Cs=inf  Measurements=off
  Mosfet1 : spsMosfetLib/Mosfet  Ron=0.1  Lon=0  Rd=0.01  Vfd=0  IC=0  Rs=1e5  Cs=inf  Measurements=off
  D : PMIOPort  Side=Left
  D1 : PMIOPort  Port=2  Side=Right
  wires:
  g/1 -> Mosfet1/1, Mosfet/1
  connections:
  Mosfet/RConn1 -- Mosfet1/RConn1
  Mosfet1/LConn1 -- D1/RConn1
  Mosfet/LConn1 -- D/RConn1

== system final_output/breaker1 ==
  g : Inport
  Mosfet : spsMosfetLib/Mosfet  Ron=0.1  Lon=0  Rd=0.01  Vfd=0  IC=0  Rs=1e5  Cs=inf  Measurements=off
  Mosfet1 : spsMosfetLib/Mosfet  Ron=0.1  Lon=0  Rd=0.01  Vfd=0  IC=0  Rs=1e5  Cs=inf  Measurements=off
  D : PMIOPort  Side=Left
  D1 : PMIOPort  Port=2  Side=Right
  wires:
  g/1 -> Mosfet/1, Mosfet1/1
  connections:
  Mosfet/LConn1 -- D/RConn1
  Mosfet1/LConn1 -- D1/RConn1
  Mosfet/RConn1 -- Mosfet1/RConn1

== system final_output/breaker2 ==
  g : Inport
  Mosfet : spsMosfetLib/Mosfet  Ron=0.1  Lon=0  Rd=0.01  Vfd=0  IC=0  Rs=1e5  Cs=inf  Measurements=off
  Mosfet1 : spsMosfetLib/Mosfet  Ron=0.1  Lon=0  Rd=0.01  Vfd=0  IC=0  Rs=1e5  Cs=inf  Measurements=off
  D : PMIOPort  Side=Left
  D1 : PMIOPort  Port=2  Side=Right
  wires:
  g/1 -> Mosfet/1, Mosfet1/1
  connections:
  Mosfet/LConn1 -- D/RConn1
  Mosfet1/LConn1 -- D1/RConn1
  Mosfet/RConn1 -- Mosfet1/RConn1

== system final_output/breaker3 ==
  g : Inport
  Mosfet : spsMosfetLib/Mosfet  Ron=0.1  Lon=0  Rd=0.01  Vfd=0  IC=0  Rs=1e5  Cs=inf  Measurements=off
  Mosfet1 : spsMosfetLib/Mosfet  Ron=0.1  Lon=0  Rd=0.01  Vfd=0  IC=0  Rs=1e5  Cs=inf  Measurements=off
  D : PMIOPort  Side=Left
  D1 : PMIOPort  Port=2  Side=Right
  wires:
  g/1 -> Mosfet1/1, Mosfet/1
  connections:
  Mosfet/RConn1 -- Mosfet1/RConn1
  Mosfet1/LConn1 -- D1/RConn1
  Mosfet/LConn1 -- D/RConn1

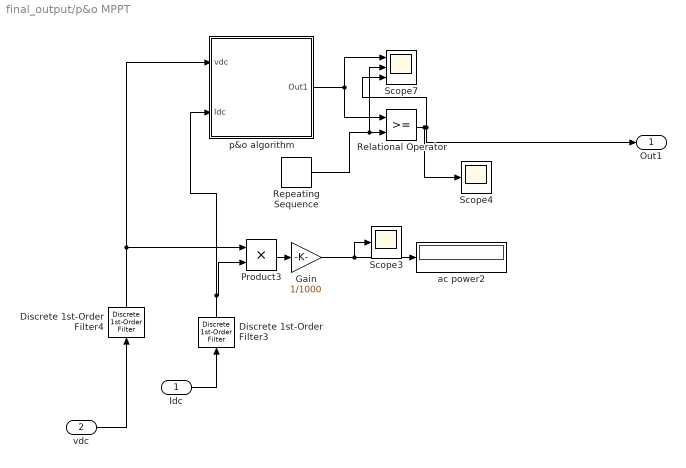
== system final_output/p&o MPPT ==
  Idc : Inport
  vdc : Inport  Port=2
  Discrete 1st-Order Filter3 : powerlib_extras/Discrete  Control Blocks/Discrete 1st-Order Filter  FilterType=Lowpass  Tc=100e-3  Ts=20e-6  Initialize=off  Vac_Init=[0.8 -25 60]  Vdc_Init=-0.4  PlotResponse=off  param1=[1 500 0.1]
  Discrete 1st-Order Filter4 : powerlib_extras/Discrete  Control Blocks/Discrete 1st-Order Filter  FilterType=Lowpass  Tc=100e-3  Ts=20e-6  Initialize=off  Vac_Init=[0.8 -25 60]  Vdc_Init=-0.4  PlotResponse=off  param1=[1 500 0.1]
  Gain : Gain  Gain=1/1000
  Product3 : Product
  Relational Operator : RelationalOperator  OutDataTypeStr=boolean  InputSameDT=off
  Repeating Sequence : simulink/Sources/Repeating Sequence  rep_seq_t="[0  1/20000]"  rep_seq_y=[0 1.2]
  Scope3 : Scope
  Scope4 : Scope
  Scope7 : Scope  NumInputPorts=3
  ac power2 : Display
  p&o algorithm : Subsystem
  Out1 : Outport
  wires:
  vdc/1 -> Discrete 1st-Order Filter4/1
  Repeating Sequence/1 -> Scope7/2, Relational Operator/2
  Gain/1 -> Scope3/1, ac power2/1
  Relational Operator/1 -> Scope4/1, Out1/1, Scope7/3
  Discrete 1st-Order Filter3/1 -> p&o algorithm/2(Idc), Product3/2
  Discrete 1st-Order Filter4/1 -> p&o algorithm/1(vdc), Product3/1
  p&o algorithm/1(Out1) -> Scope7/1, Relational Operator/1
  Product3/1 -> Gain/1
  Idc/1 -> Discrete 1st-Order Filter3/1

== system final_output/pv array 4.5KW ==
  In1 : Inport
  Constant : Constant  Value=25
  PV Array1 : spsPVArrayLib/PV Array  Npar=1  Nser=20  PlotType=array @ 25 deg.C & specified irradiances  S_vec=[1000 800 600 400 200 100]  Temp_C_vec=[ 50 ]  ModuleName=Advanced Renewable Energy AREi-230W-M6-G  PlotWhenSelected=off  Pm=230.4  Ncell=60  Voc=37.14  Isc=8  Vm=30.72  Im=7.5  beta_Voc_pc=-0.35335  alpha_Isc_pc=0.05535  beta_Voc=-0.13123  alpha_Isc=0.004428  IL=8.007  I0=2.1265e-10  nI=0.99005  Rsh=280.3446  Rs=0.2449  RobustModel=off  RobustCellTemperature=313.3991  BAL=on  Tc=1e-6  Tfilter=5e-5
      settings: AttributesFormatString=|
      | %<ModuleName>
      | %<Nser>-module string
      | %<Npar> parallel strings
  + : PMIOPort  Side=Right
  - : PMIOPort  Port=2  Side=Right
  m : Outport
  tag scope: irr=global
  wires:
  PV Array1/1 -> m/1
  Constant/1 -> PV Array1/2
  In1/1 -> PV Array1/1, [irr]
  connections:
  +/RConn1 -- PV Array1/RConn1
  PV Array1/RConn2 -- -/RConn1

== system final_output/12KW wind with p&o mppt/Subsystem ==
  In1 : Inport
  In2 : Inport  Port=2
  1\ib1 : Gain  Gain=1.732  SaturateOnIntegerOverflow=on  OutDataTypeStr=Inherit: Same as input  ParamDataTypeStr=Inherit: Same as input
  1\ib4 : Gain  Gain=1/1000  SaturateOnIntegerOverflow=on  OutDataTypeStr=Inherit: Same as input  ParamDataTypeStr=Inherit: Same as input
  Product3 : Product
  RMS : spsRMSLib/RMS  TrueRMS=on  Freq=50  RMSInit=120  Ts=50e-6
  RMS1 : spsRMSLib/RMS  TrueRMS=on  Freq=50  RMSInit=120  Ts=50e-6
  Out1 : Outport
  wires:
  In2/1 -> RMS1/1
  RMS1/1 -> Product3/2
  Product3/1 -> 1\ib4/1
  1\ib1/1 -> Product3/1
  RMS/1 -> 1\ib1/1
  1\ib4/1 -> Out1/1
  In1/1 -> RMS/1

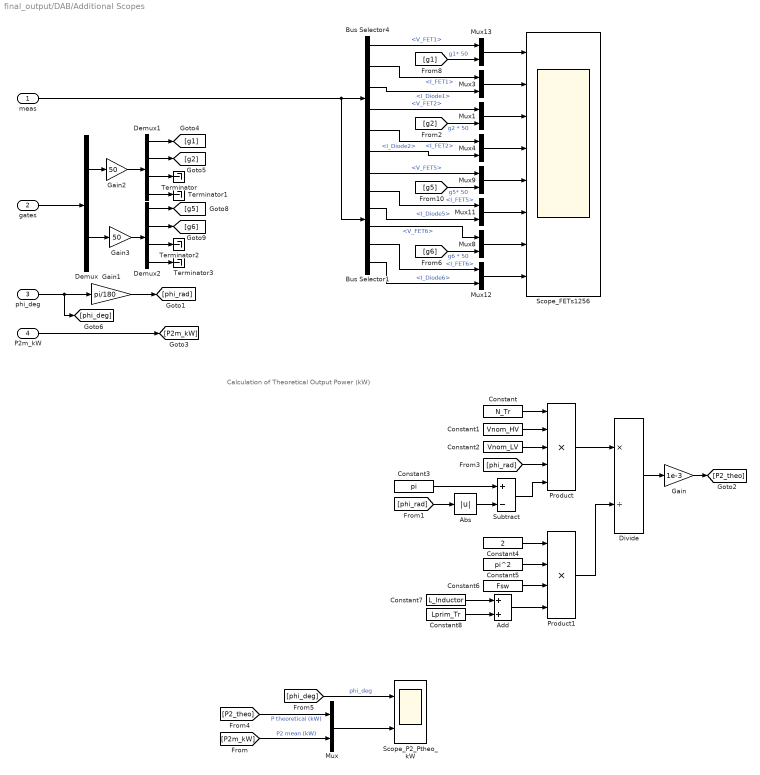
== system final_output/DAB/Additional Scopes ==
  note: Calculation of Theoretical Output Power (kW)
  meas : Inport
  gates : Inport  Port=2
  phi_deg : Inport  Port=3
  P2m_kW : Inport  Port=4
  Abs : Abs  SaturateOnIntegerOverflow=off
  Add : Sum
  Bus Selector1 : BusSelector  OutputSignals=V_FET5,I_FET5,I_Diode5,V_FET6,I_FET6,I_Diode6
  Bus Selector4 : BusSelector  OutputSignals=V_FET1,I_FET1,I_Diode1,V_FET2,I_FET2,I_Diode2
  Constant : Constant  Value=N_Tr
  Constant1 : Constant  Value=Vnom_HV
  Constant2 : Constant  Value=Vnom_LV
  Constant3 : Constant  Value=pi
  Constant4 : Constant  Value=2
  Constant5 : Constant  Value=pi^2
  Constant6 : Constant  Value=Fsw
  Constant7 : Constant  Value=L_Inductor
  Constant8 : Constant  Value=Lprim_Tr
  Demux : Demux  Outputs=[4,4]
  Demux1 : Demux
  Demux2 : Demux
  Divide : Product  Inputs=*/
  Gain : Gain  Gain=1e-3
  Gain1 : Gain  Gain=pi/180
  Gain2 : Gain  Gain=50
  Gain3 : Gain  Gain=50
  Mux{,1,3..4,8..9,11..13} (9 alike) : Mux  Inputs=2
  Product : Product  Inputs=5
  Product1 : Product  Inputs=4
  Scope_FETs1256 : Scope  NumInputPorts=8
  Scope_P2_Ptheo_kW : Scope  NumInputPorts=2
  Subtract : Sum  Inputs=+-
  Terminator{,1..3} (4 alike) : Terminator
  wires:
  gates/1 -> Demux/1
  Bus Selector4/1 -> Mux13/1  "<V_FET1>"
  [g1] -> Mux13/2  "g1* 50"
  Mux13/1 -> Scope_FETs1256/1
  [g2] -> Mux1/2  "g2 * 50"
  Bus Selector4/4 -> Mux1/1  "<V_FET2>"
  Mux3/1 -> Scope_FETs1256/2
  Bus Selector4/2 -> Mux3/1  "<I_FET1>"
  Bus Selector4/3 -> Mux3/2  "<I_Diode1>"
  Mux1/1 -> Scope_FETs1256/3
  Mux4/1 -> Scope_FETs1256/4
  Bus Selector4/5 -> Mux4/1  "<I_FET2>"
  Bus Selector4/6 -> Mux4/2  "<I_Diode2>"
  Bus Selector1/6 -> Mux12/2  "<I_Diode6>"
  Bus Selector1/5 -> Mux12/1  "<I_FET6>"
  Bus Selector1/3 -> Mux11/2  "<I_Diode5>"
  Bus Selector1/2 -> Mux11/1  "<I_FET5>"
  Bus Selector1/4 -> Mux8/1  "<V_FET6>"
  [g6] -> Mux8/2  "g6 * 50"
  [g5] -> Mux9/2  "g5* 50"
  Bus Selector1/1 -> Mux9/1  "<V_FET5>"
  Demux/1 -> Gain2/1
  Demux/2 -> Gain3/1
  Gain2/1 -> Demux1/1
  Demux1/1 -> [g1]
  Demux1/2 -> [g2]
  Demux1/3 -> Terminator/1
  Demux1/4 -> Terminator1/1
  Gain3/1 -> Demux2/1
  Demux2/1 -> [g5]
  Demux2/2 -> [g6]
  Demux2/3 -> Terminator2/1
  Demux2/4 -> Terminator3/1
  Mux9/1 -> Scope_FETs1256/5
  Mux11/1 -> Scope_FETs1256/6
  Mux8/1 -> Scope_FETs1256/7
  Mux12/1 -> Scope_FETs1256/8
  meas/1 -> Bus Selector1/1, Bus Selector4/1
  phi_deg/1 -> [phi_deg], Gain1/1
  Gain1/1 -> [phi_rad]
  Constant3/1 -> Subtract/1
  [phi_rad] -> Abs/1
  Constant/1 -> Product/1
  Constant1/1 -> Product/2
  Constant2/1 -> Product/3
  Abs/1 -> Subtract/2
  Subtract/1 -> Product/5
  Product/1 -> Divide/1
  Constant4/1 -> Product1/1
  Constant5/1 -> Product1/2
  Constant6/1 -> Product1/3
  Add/1 -> Product1/4
  Constant7/1 -> Add/1
  Constant8/1 -> Add/2
  Product1/1 -> Divide/2
  Divide/1 -> Gain/1
  P2m_kW/1 -> [P2m_kW]
  Gain/1 -> [P2_theo]
  [P2_theo] -> Mux/1  "P theoretical (kW)"
  [P2m_kW] -> Mux/2  "P2 mean (kW)"
  [phi_rad] -> Product/4
  Mux/1 -> Scope_P2_Ptheo_kW/2
  [phi_deg] -> Scope_P2_Ptheo_kW/1  "phi_deg"

== system final_output/DAB/Current Regulator ==
  Iref : Inport
  Imeas : Inport  Port=2
  PI regulator with anti-windup d1 : Subsystem  DialogController=POWERSYS.PowerSysDialog  mask(Discrete PI Controller with anti-windup){Kp=Kp_Ireg, Ki=Ki_Ireg, Par_Limits=[25, -40], Init=22, Ts=Ts_Control}
      mask prompts: Kp "Proportional gain (Kp):"; Ki "Integral gain (Ki):"; Par_Limits "Output limits: [ Upper   Lower ]"; Init "Output initial value:"; Ts "Sample time:"
      mask help: This block implements a discrete PI controller with anti-windup.
      mask init:
      | UpperLimit=Par_Limits(1);
      | LowerLimit=Par_Limits(2);
      mask Display: disp('PI');
  Sum : Sum  Inputs=|-+
  phi_deg : Outport
  wires:
  PI regulator with anti-windup d1/1(Out) -> phi_deg/1
  Imeas/1 -> Sum/1
  Iref/1 -> Sum/2
  Sum/1 -> PI regulator with anti-windup d1/1(Error)
